simulink model "BEV3EMDualFront"  (R2026b)
settings: Solver=VariableStepAuto
undefined symbols (not defined in the file): PlntDriveshftDamp, PlntDriveshftStiff, PlntEM1RotInertia, PlntEM1TransGearRatio, PlntEM1TransInInertia, PlntEM2RotInertia, PlntEM2TransGearRatio, PlntEM2TransInInertia, PlntEM3RotInertia, PlntEM3TransGearRatio, PlntEM3TransInInertia
libraries: autolibsharedcoupling x6
settings Model: ModifiedByFormat=The MathWorks, Inc.  Creator=The MathWorks, Inc.  LastModifiedBy=The MathWorks, Inc.
settings OptimizationCC: ReuseModelBlockBuffer=off
settings DebuggingCC: SubsystemReferenceDiagnosticForUnitTest=warning

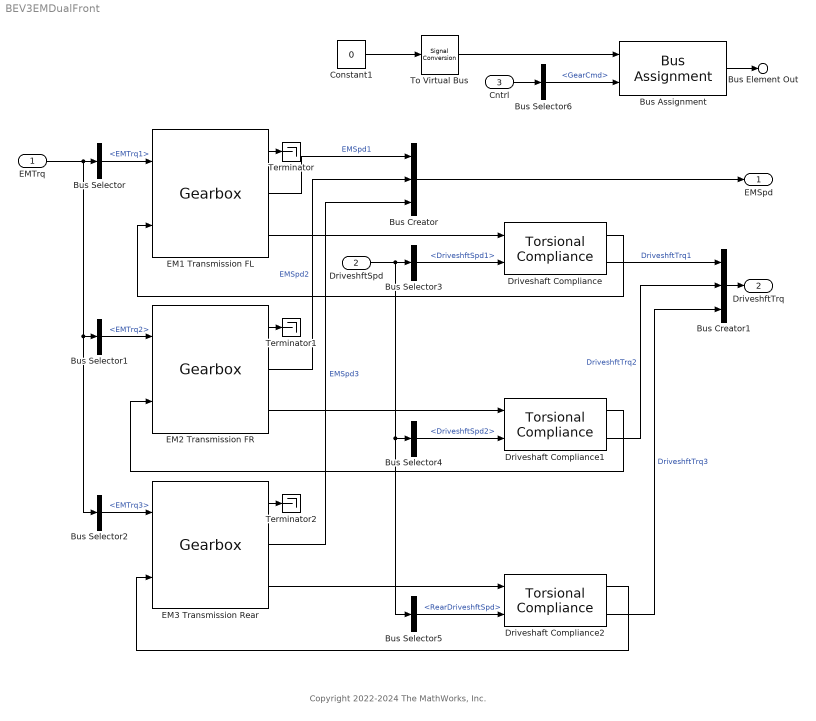
== system BEV3EMDualFront ==
  note: Copyright 2022-2024 The MathWorks, Inc.
  EMTrq : Inport
  DriveshftSpd : Inport  Port=2
  Cntrl : Inport  Port=3
  Bus Assignment : BusAssignment  AssignedSignals=Info.Trans.TransGear
  Bus Creator : BusCreator  Inputs=3
  Bus Creator1 : BusCreator  Inputs=3
  Bus Selector : BusSelector  OutputSignals=EMTrq1
  Bus Selector1 : BusSelector  OutputSignals=EMTrq2
  Bus Selector2 : BusSelector  OutputSignals=EMTrq3
  Bus Selector3 : BusSelector  OutputSignals=FrntDriveshftSpd.DriveshftSpd1
  Bus Selector4 : BusSelector  OutputSignals=FrntDriveshftSpd.DriveshftSpd2
  Bus Selector5 : BusSelector  OutputSignals=RearDriveshftSpd
  Bus Selector6 : BusSelector  OutputSignals=Trans.GearCmd
  Constant1 : Constant  Value=0  OutDataTypeStr=Bus: TransInfoBUS  SampleTime=Inf
  Driveshaft Compliance : autolibsharedcoupling/Torsional Compliance  port_config=Simulink  extInfo=off  k=PlntDriveshftStiff  b=PlntDriveshftDamp  theta_o=PlntDriveshftInitDeflect  domega_o=PlntDriveshftInitVel  omega_c=PlntDriveshftDampCutoffFreq  blkID=0  aMode=1
  Driveshaft Compliance1 : autolibsharedcoupling/Torsional Compliance  port_config=Simulink  extInfo=off  k=PlntDriveshftStiff  b=PlntDriveshftDamp  theta_o=PlntDriveshftInitDeflect  domega_o=PlntDriveshftInitVel  omega_c=PlntDriveshftDampCutoffFreq  blkID=0  aMode=1
  Driveshaft Compliance2 : autolibsharedcoupling/Torsional Compliance  port_config=Simulink  extInfo=off  k=PlntDriveshftStiff  b=PlntDriveshftDamp  theta_o=PlntDriveshftInitDeflect  domega_o=PlntDriveshftInitVel  omega_c=PlntDriveshftDampCutoffFreq  blkID=0  aMode=1
  "EM1 Transmission FL " : autolibsharedcoupling/Gearbox  port_config=Simulink  input_config=Torque input - velocity output  DiffEffModelPopup=Constant  InterpMethod=Flat  dirSwitch=on  extTamb=off  N=PlntEM1TransGearRatio  J1=PlntEM1TransInInertia + PlntEM1RotInertia  J2=PlntEM1TransOutInertia  b1=PlntEM1TransInDamp  b2=PlntEM1TransOutDamp  theta1_o=0  w1_o=PlntEM1TransInitVel  eta=PlntEM1TransEff  eta_tbl=reshape([0.64 0.76 0.8 0.81 0.83 0.84 0.84 0.56 0.73 0.78 0.8 0.83 0.84 0.84 0.54 0.71 0.77 0.8 0.82 0.84 0.84 0.53 0.71 0.77 0.8 0.83 0.84 0.84 0.51 0.71 0.77 0.8 0.83 0.84 0.85 0.52 0.7 0.77 0.8 0.83 0.84 0.85 0.51 0.71 0.76 0.79 0.83 0.84 0.85 0.5 0.69 0.76 0.79 0.82 0.84 0.85 0.45 0.68 0.75 0.78 0.82 0.84 0.85 0.43 0.67 0.74 0.78 0.81 0.83 0.84 0.38 0.63 0.71 0.75 0.8 0.82 0.83 0.81 0.86 0.88 0.89 0.89 0.89 0.9 0.77 0.85 0.87 0.88 0.89 0.9 0.9 0.72 0.82 0.86 0.87 0.88 0.89 0.9 0.68 0.8 0.84 0.86 0.88 0.89 0.89 0.67 0.8 0.84 0.86 0.88 0.89 0.9 0.67 0.8 0.84 0.86 0.88 0.89 0.9 0.65 0.8 0.84 0.86 0.88 0.89 0.9 0.64 0.79 0.83 0.86 0.88 0.89 0.9 0.63 0.78 0.83 0.86 0.88 0.89 0.9 0.59 0.76 0.82 0.85 0.87 0.89 0.9 0.53 0.73 0.8 0.83 0.86 0.88 0.89], 7, 11, 2)  Trq_bpts=[25, 50, 75, 100, 150, 200, 250]  omega_bpts=[52.4 78.5 105 131 157 183 209 262 314 419 524]  Temp_bpts=[290 358]  Tamb=297.15  blkID=0  aMode=1
      settings: LibrarySourceBlock=autolibcoupling/Gearbox
  EM2 Transmission FR : autolibsharedcoupling/Gearbox  port_config=Simulink  input_config=Torque input - velocity output  DiffEffModelPopup=Constant  InterpMethod=Flat  dirSwitch=on  extTamb=off  N=PlntEM2TransGearRatio  J1=PlntEM2TransInInertia + PlntEM2RotInertia  J2=PlntEM2TransOutInertia  b1=PlntEM2TransInDamp  b2=PlntEM2TransOutDamp  theta1_o=0  w1_o=PlntEM2TransInitVel  eta=PlntEM2TransEff  eta_tbl=reshape([0.64 0.76 0.8 0.81 0.83 0.84 0.84 0.56 0.73 0.78 0.8 0.83 0.84 0.84 0.54 0.71 0.77 0.8 0.82 0.84 0.84 0.53 0.71 0.77 0.8 0.83 0.84 0.84 0.51 0.71 0.77 0.8 0.83 0.84 0.85 0.52 0.7 0.77 0.8 0.83 0.84 0.85 0.51 0.71 0.76 0.79 0.83 0.84 0.85 0.5 0.69 0.76 0.79 0.82 0.84 0.85 0.45 0.68 0.75 0.78 0.82 0.84 0.85 0.43 0.67 0.74 0.78 0.81 0.83 0.84 0.38 0.63 0.71 0.75 0.8 0.82 0.83 0.81 0.86 0.88 0.89 0.89 0.89 0.9 0.77 0.85 0.87 0.88 0.89 0.9 0.9 0.72 0.82 0.86 0.87 0.88 0.89 0.9 0.68 0.8 0.84 0.86 0.88 0.89 0.89 0.67 0.8 0.84 0.86 0.88 0.89 0.9 0.67 0.8 0.84 0.86 0.88 0.89 0.9 0.65 0.8 0.84 0.86 0.88 0.89 0.9 0.64 0.79 0.83 0.86 0.88 0.89 0.9 0.63 0.78 0.83 0.86 0.88 0.89 0.9 0.59 0.76 0.82 0.85 0.87 0.89 0.9 0.53 0.73 0.8 0.83 0.86 0.88 0.89], 7, 11, 2)  Trq_bpts=[25, 50, 75, 100, 150, 200, 250]  omega_bpts=[52.4 78.5 105 131 157 183 209 262 314 419 524]  Temp_bpts=[290 358]  Tamb=297.15  blkID=0  aMode=1
      settings: LibrarySourceBlock=autolibcoupling/Gearbox
  EM3 Transmission Rear : autolibsharedcoupling/Gearbox  port_config=Simulink  input_config=Torque input - velocity output  DiffEffModelPopup=Constant  InterpMethod=Flat  dirSwitch=on  extTamb=off  N=PlntEM3TransGearRatio  J1=PlntEM3TransInInertia + PlntEM3RotInertia  J2=PlntEM3TransOutInertia  b1=PlntEM3TransInDamp  b2=PlntEM3TransOutDamp  theta1_o=0  w1_o=PlntEM3TransInitVel  eta=PlntEM3TransEff  eta_tbl=reshape([0.64 0.76 0.8 0.81 0.83 0.84 0.84 0.56 0.73 0.78 0.8 0.83 0.84 0.84 0.54 0.71 0.77 0.8 0.82 0.84 0.84 0.53 0.71 0.77 0.8 0.83 0.84 0.84 0.51 0.71 0.77 0.8 0.83 0.84 0.85 0.52 0.7 0.77 0.8 0.83 0.84 0.85 0.51 0.71 0.76 0.79 0.83 0.84 0.85 0.5 0.69 0.76 0.79 0.82 0.84 0.85 0.45 0.68 0.75 0.78 0.82 0.84 0.85 0.43 0.67 0.74 0.78 0.81 0.83 0.84 0.38 0.63 0.71 0.75 0.8 0.82 0.83 0.81 0.86 0.88 0.89 0.89 0.89 0.9 0.77 0.85 0.87 0.88 0.89 0.9 0.9 0.72 0.82 0.86 0.87 0.88 0.89 0.9 0.68 0.8 0.84 0.86 0.88 0.89 0.89 0.67 0.8 0.84 0.86 0.88 0.89 0.9 0.67 0.8 0.84 0.86 0.88 0.89 0.9 0.65 0.8 0.84 0.86 0.88 0.89 0.9 0.64 0.79 0.83 0.86 0.88 0.89 0.9 0.63 0.78 0.83 0.86 0.88 0.89 0.9 0.59 0.76 0.82 0.85 0.87 0.89 0.9 0.53 0.73 0.8 0.83 0.86 0.88 0.89], 7, 11, 2)  Trq_bpts=[25, 50, 75, 100, 150, 200, 250]  omega_bpts=[52.4 78.5 105 131 157 183 209 262 314 419 524]  Temp_bpts=[290 358]  Tamb=297.15  blkID=0  aMode=1
      settings: LibrarySourceBlock=autolibcoupling/Gearbox
  Terminator : Terminator
  Terminator1 : Terminator
  Terminator2 : Terminator
  To Virtual Bus : SignalConversion  ConversionOutput=Virtual bus  OverrideOpt=off
  EMSpd : Outport  VectorParamsAs1DForOutWhenUnconnected=off  BusOutputAsStruct=on
  DriveshftTrq : Outport  Port=2  VectorParamsAs1DForOutWhenUnconnected=off
  Bus Element Out : Outport  Port=3  PortName=TransInfo
  wires:
  Bus Creator/1 -> EMSpd/1
  Bus Selector1/1 -> EM2 Transmission FR/1  "<EMTrq2>"
  Bus Selector/1 -> "EM1 Transmission FL "/1  "<EMTrq1>"
  Bus Creator1/1 -> DriveshftTrq/1
  Driveshaft Compliance1/2 -> Bus Creator1/2  "DriveshftTrq2"
  Bus Selector3/1 -> Driveshaft Compliance/2  "<DriveshftSpd1>"
  EM2 Transmission FR/3 -> Driveshaft Compliance1/1
  Driveshaft Compliance/2 -> Bus Creator1/1  "DriveshftTrq1"
  EMTrq/1 -> Bus Selector2/1, Bus Selector1/1, Bus Selector/1
  Driveshaft Compliance/1 -> "EM1 Transmission FL "/2
  Driveshaft Compliance1/1 -> EM2 Transmission FR/2
  "EM1 Transmission FL "/3 -> Driveshaft Compliance/1
  Bus Selector4/1 -> Driveshaft Compliance1/2  "<DriveshftSpd2>"
  Bus Selector5/1 -> Driveshaft Compliance2/2  "<RearDriveshftSpd>"
  Driveshaft Compliance2/1 -> EM3 Transmission Rear/2
  DriveshftSpd/1 -> Bus Selector4/1, Bus Selector5/1, Bus Selector3/1
  EM3 Transmission Rear/3 -> Driveshaft Compliance2/1
  Driveshaft Compliance2/2 -> Bus Creator1/3  "DriveshftTrq3"
  Bus Selector2/1 -> EM3 Transmission Rear/1  "<EMTrq3>"
  "EM1 Transmission FL "/2 -> Bus Creator/1  "EMSpd1"
  EM2 Transmission FR/2 -> Bus Creator/2  "EMSpd2"
  EM3 Transmission Rear/2 -> Bus Creator/3  "EMSpd3"
  "EM1 Transmission FL "/1 -> Terminator/1
  EM2 Transmission FR/1 -> Terminator1/1
  EM3 Transmission Rear/1 -> Terminator2/1
  Cntrl/1 -> Bus Selector6/1
  Bus Selector6/1 -> Bus Assignment/2  "<GearCmd>"
  To Virtual Bus/1 -> Bus Assignment/1
  Bus Assignment/1 -> Bus Element Out/1
  Constant1/1 -> To Virtual Bus/1
